simulink model "Lift"  (R2020a)
settings: Solver=VariableStepAuto  StartTime=0.0  StopTime=10.0  RelTol=1e-3
settings Model: Creator=Hp  LastModifiedBy=Hp

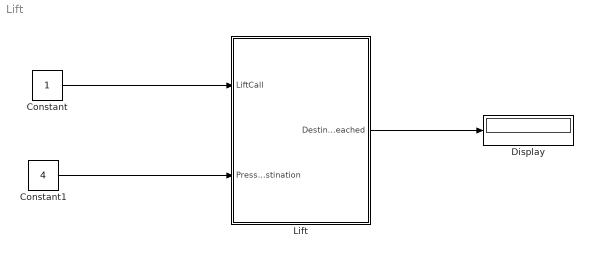
== system Lift ==
  Constant : Constant
  Constant1 : Constant  Value=4
  Display : Display
  Lift : Stateflow chart  TreatAsAtomicUnit=on
  wires:
  Constant/1 -> Lift/1(LiftCall)
  Constant1/1 -> Lift/2(PressedDestination)
  Lift/1(DestinationReached) -> Display/1

== stateflow chart Lift/Lift ==
  state StopState
    state Stopped_and_Waiting
      state InitialState
        en:
        Motor=0; Brake=1;
        Command=0;
        Door=0;
      state DestinationSelection
        en:
        Destination=PressedDestination;
      state CommandMade
        en:
        command=1;
      state SettingDown
        en:
        Up=0;
      state SettingUp
        en:
        Up=1;
      (default) -> InitialState
      InitialState -> DestinationSelection : [LiftCall==1]
      DestinationSelection -> SettingDown [order 2] : [checkPosition(CurrentPos,Destination)==-1]
      DestinationSelection -> SettingUp [order 1] : [checkPosition(CurrentPos,Destination)==1]
      SettingUp -> CommandMade
      SettingDown -> CommandMade
    state Stopped_at_Destination
      (default) -> (junction 113) : % DoorOpening
      (junction 113) -> (junction 114) [order 1] : [checkPosition(CurrentPos,Destination)==0]
      (junction 113) -> (junction 115) [order 2] : {Door=0;}
      (junction 114) -> (junction 116) : {Door=1;DestinationReached=CurrentPos;}
      (junction 116) -> (junction 115)
      (junction 115) -> (junction 117)
    (default) -> Stopped_and_Waiting
    Stopped_and_Waiting -> Stopped_and_Waiting : [LiftCall==0&&Command==0]
    Stopped_at_Destination -> Stopped_and_Waiting : [Door==1]
    DestinationSelection -> Stopped_at_Destination [order 3] : [checkPosition(CurrentPos,Destination)==0]
  state MovingState
    state MotorOn
      en:
      Motor=1;Brake=0;
      Door=0
    state MoveDown
      en:
      CurrentPos = CurrentPos - 1;
    state MoveUp
      en:
      CurrentPos = CurrentPos + 1;
    (default) -> MotorOn
    MotorOn -> MoveDown [order 2] : [Up==0]
    MotorOn -> MoveUp [order 1] : [Up==1]
    MoveDown -> MoveDown : [checkPosition(CurrentPos,Destination)==-1]
    MoveUp -> MoveUp : [checkPosition(CurrentPos,Destination)==1]
  (default) -> StopState : {CurrentPos=0;}
  MovingState -> Stopped_at_Destination : [CurrentPos==Destination]
  CommandMade -> MovingState : [command==1]
  data: CPos function_input; pos function_output; Destn function_input; LiftCall input; PressedDestination input; Command local; CurrentPos local =0; Destination local; Door local; Up local; command local; Brake local; Motor local; DestinationReached output
  function pos=checkPosition(CPos,Destn):
    | function pos=checkPosition(CPos,Destn)
    |      if(CPos==Destn)
    |         pos=0;
    |       else if(CPos>Destn)
    |             pos=-1;
    |       else 
    |                 pos=1;
    |      end
    | end
